simulink model "position_interface_astar"  (R2019b)
settings: Solver=FixedStepAuto  StartTime=0.0  StopTime=Inf  FixedStep=FIXED_STEP_SIZE  RelTol=1e-3
values from neighbouring files (symbols this model uses):
  GAZEBO_SYNC_DT = 0.01    [position_interface_main.m]
undefined symbols (not defined in the file or in its folder): Angular, Linear
libraries: robotlib x4, robotgazebolib x1
settings Model: SimulationMode=external  Creator=ananda  LastModifiedBy=theis
settings OptimizationCC: EnhancedBackFolding=on  PassReuseOutputArgsAs=Individual arguments  ZeroExternalMemoryAtStartup=off  ZeroInternalMemoryAtStartup=off  MaxStackSize=64  OptimizeBlockOrder=speed  DifferentSizesBufferReuse=on  OptimizationCustomize=off  EfficientTunableParamExpr=on
settings DebuggingCC: ParameterTunabilityLossMsg=error
settings HardwareCC: ProdBitPerPointer=32  ProdBitPerSizeT=32  ProdBitPerPtrDiffT=32  ProdLargestAtomicFloat=None  ProdIntDivRoundTo=Undefined  ProdEndianess=Unspecified  ProdWordSize=32  ProdHWDeviceType=Generic->Unspecified (assume 32-bit Generic)  UseEmbeddedCoderFeatures=off
settings SFSimCC: MATLABDynamicMemAlloc=off
settings RTWCC: SystemTargetFile=ert.tlc  HardwareBoard=Robot Operating System (ROS)  TLCOptions="-aInlineSetEventsForThisBaseRateFcn=TLC_FALSE -aSuppressMultiTaskScheduler=TLC_FALSE  -aRateBasedStepFcn=0"  TemplateMakefile=ert_default_tmf  GenerateReport=on  Toolchain=Catkin  IncludeHyperlinkInReport=on  LaunchReport=on  TargetLang=C++  GenerateTraceInfo=on  GenerateTraceReport=on  GenerateTraceReportSl=on  GenerateTraceReportSf=on  GenerateTraceReportEml=on
settings CodeAppCC: ForceParamTrailComments=on  IgnoreCustomStorageClasses=off  OperatorAnnotations=on  SimulinkDataObjDesc=on  SFDataObjDesc=on  InsertBlockDesc=on
settings ERTTargetCC: SupportNonInlinedSFcns=on

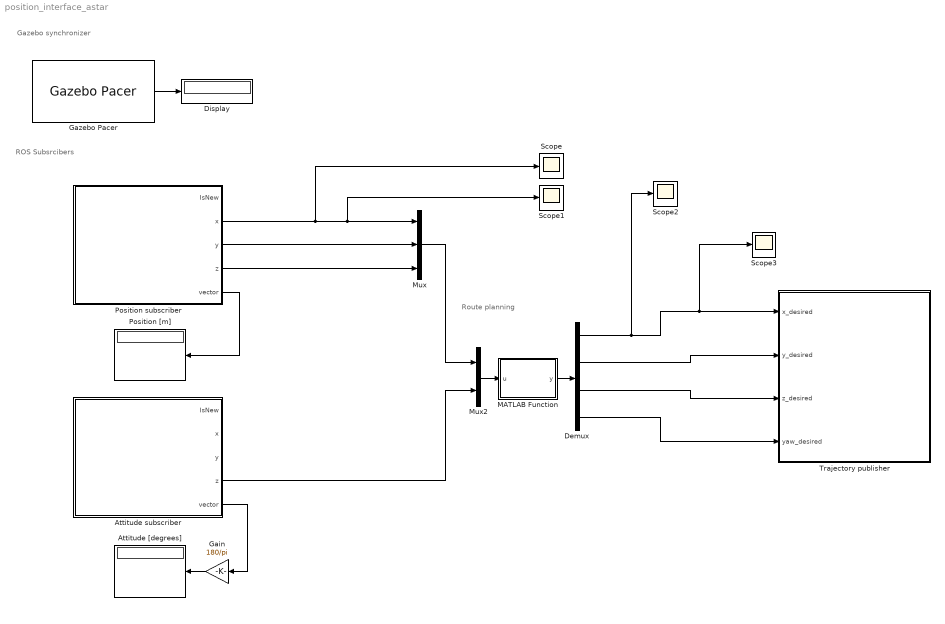
== system position_interface_astar ==
  note: Gazebo synchronizer
  note: ROS Subsrcibers
  note: Route planning
  Attitude [degrees] : Display
  Attitude subscriber : Subsystem
  Demux : Demux
  Display : Display
  Gain : Gain  Gain=180/pi
  Gazebo Pacer : robotgazebolib/Gazebo Pacer  ResetBehavior=Reset Gazebo simulation time  SampleTime=GAZEBO_SYNC_DT
      settings: SourceProductName=Robotics System Toolbox  SourceProductBaseCode=RO
  MATLAB Function : MATLAB Function  TreatAsAtomicUnit=on
  Mux : Mux  Inputs=3
  Mux2 : Mux  Inputs=2
  Position [m] : Display
  Position subscriber : Subsystem
  Scope{,1..3} (4 alike) : Scope
  Trajectory publisher : Subsystem
  wires:
  Position subscriber/5(vector) -> Position [m]/1
  Attitude subscriber/5(vector) -> Gain/1
  Gain/1 -> Attitude [degrees]/1
  Gazebo Pacer/1 -> Display/1
  MATLAB Function/1(y) -> Demux/1
  Mux2/1 -> MATLAB Function/1(u)
  Mux/1 -> Mux2/1
  Demux/4 -> Trajectory publisher/4(yaw_desired)
  Position subscriber/3(y) -> Mux/2
  Demux/2 -> Trajectory publisher/2(y_desired)
  Position subscriber/2(x) -> Scope/1, Scope1/1, Mux/1
  Attitude subscriber/4(z) -> Mux2/2
  Demux/1 -> Scope2/1, Scope3/1, Trajectory publisher/1(x_desired)
  Position subscriber/4(z) -> Mux/3
  Demux/3 -> Trajectory publisher/3(z_desired)

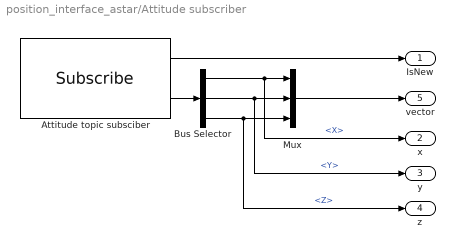
== system position_interface_astar/Attitude subscriber ==
  Attitude topic subsciber : robotlib/Subscribe  topicSource=Specify your own  topic=/hummingbird/orientation_rpy  messageType=geometry_msgs/Vector3  sampleTime=ATTI_SUB_DT  messageQueueLength=1
      settings: SourceProductName=ROS Toolbox
  Bus Selector : BusSelector  OutputSignals=X,Y,Z
  Mux : Mux  Inputs=3
  IsNew : Outport
  x : Outport  Port=2
  y : Outport  Port=3
  z : Outport  Port=4
  vector : Outport  Port=5
  wires:
  Bus Selector/3 -> z/1, Mux/3  "<Z>"
  Bus Selector/2 -> y/1, Mux/2  "<Y>"
  Bus Selector/1 -> x/1, Mux/1  "<X>"
  Attitude topic subsciber/2 -> Bus Selector/1
  Attitude topic subsciber/1 -> IsNew/1
  Mux/1 -> vector/1

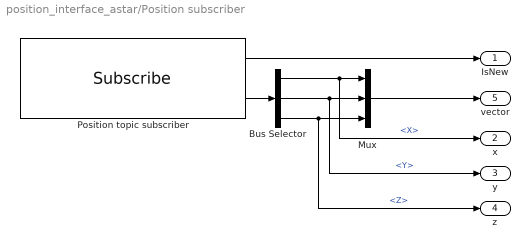
== system position_interface_astar/Position subscriber ==
  Bus Selector : BusSelector  OutputSignals=Point.X,Point.Y,Point.Z
  Mux : Mux  Inputs=3
  Position topic subscriber : robotlib/Subscribe  topicSource=Specify your own  topic=/hummingbird/odometry_sensor1/position  messageType=geometry_msgs/PointStamped  sampleTime=POS_SUB_DT  messageQueueLength=1
      settings: SourceProductName=ROS Toolbox
  IsNew : Outport
  x : Outport  Port=2
  y : Outport  Port=3
  z : Outport  Port=4
  vector : Outport  Port=5
  wires:
  Bus Selector/3 -> z/1, Mux/3  "<Z>"
  Bus Selector/2 -> y/1, Mux/2  "<Y>"
  Mux/1 -> vector/1
  Bus Selector/1 -> x/1, Mux/1  "<X>"
  Position topic subscriber/2 -> Bus Selector/1
  Position topic subscriber/1 -> IsNew/1

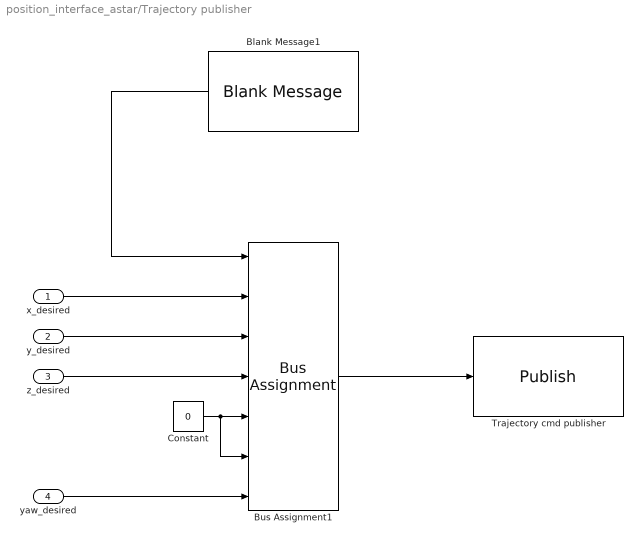
== system position_interface_astar/Trajectory publisher ==
  x_desired : Inport
  y_desired : Inport  Port=2
  z_desired : Inport  Port=3
  yaw_desired : Inport  Port=4
  Blank Message1 : robotlib/Blank Message  messageClass=Message  entityType=geometry_msgs/Twist  messageType=geometry_msgs/Twist  SampleTime=inf
      settings: SourceProductName=ROS Toolbox
  Bus Assignment1 : BusAssignment  AssignedSignals=Linear.X,Linear.Y,Linear.Z,Angular.X,Angular.Y,Angular.Z
  Constant : Constant  Value=0
  Trajectory cmd publisher : robotlib/Publish  topicSource=Specify your own  topic=/matlab/tracejtoryTwist  messageType=geometry_msgs/Twist  messageQueueLength=1
      settings: SourceProductName=ROS Toolbox
  wires:
  Blank Message1/1 -> Bus Assignment1/1
  Constant/1 -> Bus Assignment1/6, Bus Assignment1/5
  Bus Assignment1/1 -> Trajectory cmd publisher/1
  x_desired/1 -> Bus Assignment1/2
  y_desired/1 -> Bus Assignment1/3
  z_desired/1 -> Bus Assignment1/4
  yaw_desired/1 -> Bus Assignment1/7

== matlab function position_interface_astar/MATLAB Function ==
  data: u input; y output; route_2d parameter
function y = fcn(u, route_2d)

persistent count;

if (isempty(count))
    count = 0;
end

% yaw_ref = [0; 90; 180; -90; 0; 0]*pi/180;
yaw_ref = zeros(1,length(route_2d)).';

idx = mod(count,length(yaw_ref)) + 1;

posdiff = norm(route_2d(:,idx)-u(1:3));

% yawdiff = yaw_ref(idx) - u(4);
% yawdiff = atan2(sin(yawdiff), cos(yawdiff));
% 
% if idx == length(route)
%     yawdiff = 0;
% end

if count < length(route_2d)-1
    if posdiff < 0.10 %&& abs(yawdiff) < 5*pi/180
        count = count + 1;
        idx = mod(count,length(yaw_ref)) + 1;
    end
end

y = [route_2d(:, idx); yaw_ref(idx)];
